simulink model "controller_ballcatcher_overdo"  (R2018b)
settings: Solver=FixedStepDiscrete  StartTime=0.0  StopTime=10.0  FixedStep=param_controller.T_a  RelTol=1e-3
InitFcn:
  | iiwa_joint_trajectoryfollowingcontrol_rigid_parameters;
values from neighbouring files (symbols this model uses):
  estimator_init_struct = struct()    [init_estimator_struct.m]
  filter_tau_p_slow_T_1 = filter_tau_slow_T_1    [parameters.m]
  filter_tau_p_T_1 = filter_tau_T_1    [parameters.m]
  filter_tau_slow_T_1 = 1./(2*pi*[200;200;200;200;200;200;200])    [parameters.m]
  filter_tau_T_1 = 1./(2*pi*[400;400;400;400;500;1000;1000])    [parameters.m]
  filter_theta_p_slow_T_1 = filter_tau_slow_T_1    [parameters.m]
  filter_theta_p_T_1 = filter_tau_T_1    [parameters.m]
  filter_theta_slow_T_1 = filter_tau_slow_T_1    [parameters.m]
  height_of_catch = 0.9    [init_estimator_struct.m]
  optitrack_data = struct()    [init_parabola.m]
  param_nullspace = struct()    [parameters.m]
  param_robot = struct()    [parameters.m]
  positions = struct()    [init_common_positions.m]
  sensor_torque_offset = [0.53;-0.095;-0.189;0.07;-0.058;0.0025;-0.12]    [parameters.m]
  timing = struct()    [parameters.m]
undefined symbols (not defined in the file or in its folder): param_controller
libraries: simulink_extras x1
(part 1 of 2)
settings Model: TCT_ExtModeMexArgs=[128 131 86 77 1 1],16842784  SimulationMode=external  Creator=cha  LastModifiedBy=user
settings SolverCC: AutoInsertRateTranBlk=on
settings DataIOCC: LoggingToFile=on  LoggingFileName=benniii.mat
settings OptimizationCC: UseFloatMulNetSlope=on  PassReuseOutputArgsThreshold=0  LocalBlockOutputs=off  EfficientFloat2IntCast=on  OptimizeBlockOrder=speed  DifferentSizesBufferReuse=on
settings DebuggingCC: ParameterTunabilityLossMsg=error
settings HardwareCC: ProdLongLongMode=on
settings ModelReferenceCC: EnableParallelModelReferenceBuilds=on  ModelReferenceNumInstancesAllowed=Single
settings SFSimCC: SimUseLocalCustomCode=off  MATLABDynamicMemAlloc=off
settings RTWCC: SystemTargetFile=TwinCAT.tlc  GenCodeOnly=on  MakeCommand=make_tct  TemplateMakefile=tct_msbuild.tmf  Description=TwinCAT Target  GenerateReport=on  RTWUseLocalCustomCode=off  TargetLang=C++
settings RTWCC: CustomHeaderCode=|
  | #define fflush(stdout)
  | #define printf(...) m_spSrv->TcReportLog(ADSLOG_MSGTYPE_LOG,__VA_ARGS__)
settings CodeAppCC: ForceParamTrailComments=on  MaxIdLength=47  OperatorAnnotations=on  StateflowObjectComments=on  MATLABSourceComments=on
settings STFCustomTargetCC: TargetLangStandard=C++03 (ISO)  CompOptLevelCompliant=on  MATLABClassNameForMDSCustomization=Simulink.SoftwareTarget.TargetSpecificTriggerConfigurationBase  GRTInterface=on  SystemTargetFile=TwinCAT.tlc

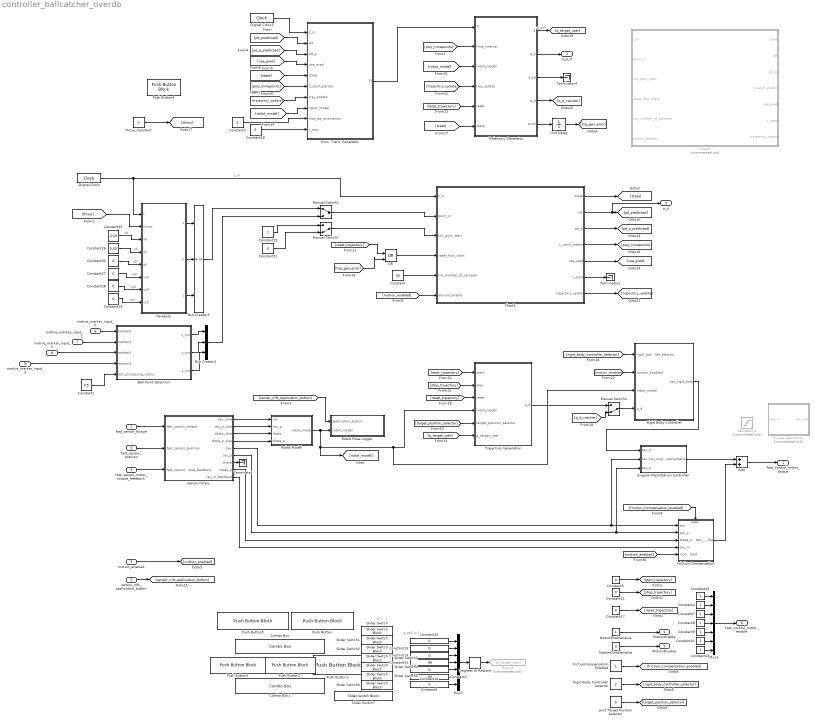
== system controller_ballcatcher_overdo ==
  note: O
  note: q_soll in °
  note: I
  fast_sensor_torque : Inport
  fast_sensor_position : Inport  Port=2
  fast_sensor_motor_torque_feedback : Inport  Port=3
  motion_enabled : Inport  Port=4
  sensor_mft_application_button : Inport  Port=5
  motive_marker_input_0 : Inport  Port=6  OutDataTypeStr=Bus: Marker
  motive_marker_input_1 : Inport  Port=7  OutDataTypeStr=Bus: Marker
  motive_marker_input_2 : Inport  Port=8  OutDataTypeStr=Bus: Marker
  motive_marker_input_3 : Inport  Port=9  OutDataTypeStr=Bus: Marker
  Add : Sum
  Ball Point Selection : MATLAB Function  TreatAsAtomicUnit=on
  Bus Creator1 : BusCreator  Inputs=3
  Bus Creator3 : BusCreator  Inputs=3
  Chart1 : Stateflow chart  TreatAsAtomicUnit=on
  Chart3 : Subsystem  Commented=on
      mask help: Simulink:masks:GenSFuncDesc_MD
      mask Help: eval('feval(''rtwprivate'',''rtwhelpview'',''rtw_sfcn_block'')');
  Combo Box : ComboBox  WebBlockId=803  SelectedLabel=2: Joint-based E/A Linearization
      settings: Values={{'1: Gravity Compensation q-based', '2: Joint-based E/A Linearization'}, [1 2]}
  Combo Box1 : ComboBox  WebBlockId=804  SelectedLabel=0: Candle position
      settings: Values={{'0: Candle position', '1: User defined position'}, [0 1]}
  Constant : Constant  Value=50
  Constant1 : Constant  Value=3.5
  Constant{4,7..10,19,22..23} (8 alike) : Constant
  Constant{3,5..6,11..14,16..17,21,27..30} (14 alike) : Constant  Value=0
  Constant15 : Constant  Value=-90
  Constant18 : Constant  Value=5
  Constant2 : Constant  Value=-90
  Constant25 : Constant  Value=-0.05
  Constant26 : Constant  Value=0.35
  Degrees to Radians : simulink_extras/Transformations/Degrees to Radians
  Digital Clock : DigitalClock  SampleTime=timing.T_optitrack
  Digital Clock1 : DigitalClock  SampleTime=timing.T_iiwa
  FictionCompensationEnabled : Constant
  Friction Compensation : Subsystem
  Goto11 : Goto  Commented=on  GotoTag=q_target_user
  Hom. Trans. Generator : MATLAB Function  TreatAsAtomicUnit=on
  Joint Target Position Selector : Constant  Value=0  OutDataTypeStr=uint32
  Manual Switch2 : ManualSwitch
  Manual Switch4 : ManualSwitch  CurrentSetting=0
  Manual Switch7 : ManualSwitch  CurrentSetting=0
  MotionDisableValue : Constant  Value=0
  MotionEnableValue : Constant
  Mux1 : Mux  Inputs=7
  Mux3 : Mux  Inputs=7
  OR : Logic  Operator=OR  IconShape=distinctive  AllPortsSameDT=off  OutDataTypeStr=boolean
  Parabola : MATLAB Function  TreatAsAtomicUnit=on
  Push Button : PushButtonBlock  WebBlockId=1354  ButtonText=Motion disable
  Push Button1 : PushButtonBlock  WebBlockId=1355  ButtonText=Reset Trajectory
  Push Button2 : PushButtonBlock  WebBlockId=1030  ButtonText=Stop trajectory
  Push Button3 : PushButtonBlock  WebBlockId=1026  ButtonText=Start trajectory
  Push Button4 : PushButtonBlock  WebBlockId=2019  ButtonText=Throw
  Push Button5 : PushButtonBlock  WebBlockId=1353  ButtonText=Motion enable
  Rigid Body Controller : Subsystem
  Rigid Body Controller Selector : Constant  Value=2  OutDataTypeStr=uint32
  Robot Model : MATLAB Function  TreatAsAtomicUnit=on
  Robot Pose Logger : MATLAB Function  TreatAsAtomicUnit=on
  Saturation1 : Saturate  Commented=on  UpperLimit=param_robot.tau_saturation_max  LowerLimit=-param_robot.tau_saturation_max
  Sensor Filters : Subsystem
  Singular Perturbation Controller : MATLAB Function  TreatAsAtomicUnit=on
  Slider Switch : SliderSwitchBlock  WebBlockId=1027  LabelPosition=Hide
      settings: Values={{'Axis1', ''}, [0 1]}
  Slider Switch1 : SliderSwitchBlock  WebBlockId=1029  LabelPosition=Hide
      settings: Values={{'Axis2', ''}, [0 1]}
  Slider Switch2 : SliderSwitchBlock  WebBlockId=1031  LabelPosition=Hide
      settings: Values={{'Axis3', ''}, [0 1]}
  Slider Switch3 : SliderSwitchBlock  WebBlockId=1022  LabelPosition=Hide
      settings: Values={{'Axis4', ''}, [0 1]}
  Slider Switch4 : SliderSwitchBlock  WebBlockId=1028  LabelPosition=Hide
      settings: Values={{'Axis5', ''}, [0 1]}
  Slider Switch5 : SliderSwitchBlock  WebBlockId=1025  LabelPosition=Hide
      settings: Values={{'Axis6', ''}, [0 1]}
  Slider Switch6 : SliderSwitchBlock  WebBlockId=1021  LabelPosition=Hide
      settings: Values={{'Axis7', ''}, [0 1]}
  Slider Switch7 : SliderSwitchBlock  WebBlockId=1032  LabelPosition=Hide
      settings: Values={{'Friction Compensation', ''}, [0 1]}
  Terminator : Terminator
  Terminator1 : Terminator
  Terminator4 : Terminator
  Throw_Constant : Constant  Value=0
  Torque Saturation1 : MATLAB Function  Commented=on  TreatAsAtomicUnit=on
  Trajectory Generation : Subsystem
  Trajectory Generator : MATLAB Function  TreatAsAtomicUnit=on
  Unit Delay : UnitDelay  SampleTime=-1
  fast_control_motor_torque : Outport
  q_p_d : Outport  Port=2  VectorParamsAs1DForOutWhenUnconnected=on
  p_d : Outport  Port=3  VectorParamsAs1DForOutWhenUnconnected=on
  MotionEnable : Outport  Port=4
  MotionDisable : Outport  Port=5
  fast_control_motor_enable : Outport  Port=6
  wires:
  MotionEnableValue/1 -> MotionEnable/1
  motion_enabled/1 -> [motion_enabled]
  MotionDisableValue/1 -> MotionDisable/1
  Sensor Filters/5(tau) -> Singular Perturbation Controller/2(tau), Friction Compensation/1(tau)
  Mux1/1 -> fast_control_motor_enable/1
  Constant22/1 -> Mux1/1
  Constant4/1 -> Mux1/2
  Constant7/1 -> Mux1/3
  Constant8/1 -> Mux1/4
  Constant9/1 -> Mux1/5
  Constant10/1 -> Mux1/6
  Constant23/1 -> Mux1/7
  fast_sensor_torque/1 -> Sensor Filters/1(fast_sensor_torque)
  fast_sensor_position/1 -> Sensor Filters/2(fast_sensor_position)
  fast_sensor_motor_torque_feedback/1 -> Sensor Filters/3(fast_sensor_motor_torque_feedback)
  Sensor Filters/9(tau_m_feedback) -> Friction Compensation/4(tau_m)
  Sensor Filters/6(tau_p) -> Singular Perturbation Controller/3(tau_p), Friction Compensation/2(tau_p)
  Sensor Filters/8(theta_p) -> Friction Compensation/3(theta_p)
  Friction Compensation/1(tau_fm_hat) -> Add/2
  Constant5/1 -> [start_trajectory]
  [motion_enabled] -> Friction Compensation/5(motion_enabled)
  Rigid Body Controller Selector/1 -> [rigid_body_controller_selector]
  FictionCompensationEnabled/1 -> [friction_compensation_enabled]
  [friction_compensation_enabled] -> Friction Compensation/Enable
  Sensor Filters/7(theta) -> Terminator/1
  Joint Target Position Selector/1 -> [target_position_selector]
  Constant6/1 -> Mux3/7
  Constant12/1 -> Mux3/1
  Constant16/1 -> Mux3/5
  Mux3/1 -> Degrees to Radians/1
  Constant15/1 -> Mux3/4
  Constant13/1 -> Mux3/2
  Constant2/1 -> Mux3/6
  Constant14/1 -> Mux3/3
  Constant11/1 -> [stop_trajectory]
  sensor_mft_application_button/1 -> [sensor_mft_application_button]
  Degrees to Radians/1 -> Goto11/1
  Sensor Filters/1(tau_slow) -> Robot Model/1(tau)
  Sensor Filters/2(tau_p_slow) -> Robot Model/2(tau_p)
  Sensor Filters/3(theta_slow) -> Robot Model/3(theta)
  Sensor Filters/4(theta_p_slow) -> Robot Model/4(theta_p)
  [sensor_mft_application_button] -> Robot Pose Logger/1(application_button)
  Robot Model/1(robot_model) -> Rigid Body Controller/3(robot_model), Trajectory Generation/4(robot_model), [robot_model], Robot Pose Logger/2(robot_model)
  Trajectory Generator/1(q) -> [q_target_user]  "q_soll"
  [use_pred] -> Hom. Trans. Generator/4(use_pred)
  [pd_p_predicted] -> Hom. Trans. Generator/3(pd_p)
  [state] -> Hom. Trans. Generator/5(state)
  Trajectory Generator/2(q_p) -> q_p_d/1
  [pd_predicted] -> Hom. Trans. Generator/2(pd)
  Constant21/1 -> Manual Switch7/2
  Constant19/1 -> Manual Switch7/1
  Digital Clock1/1 -> Hom. Trans. Generator/1(t_in)
  motive_marker_input_0/1 -> Ball Point Selection/1(marker0)
  [q_target_user] -> Trajectory Generation/6(q_target_user)
  [reset_trajectory] -> Trajectory Generation/3(reset)
  [stop_trajectory] -> Trajectory Generation/2(stop)
  [target_position_selector] -> Trajectory Generation/5(target_position_selector)
  [rigid_body_controller_selector] -> Rigid Body Controller/1(rigid_body_controller_selector)
  [start_trajectory] -> Trajectory Generation/1(start)
  [motion_enabled] -> Rigid Body Controller/2(motion_enabled)
  [robot_model] -> Trajectory Generator/3(robot_model)
  Singular Perturbation Controller/1(tau_singularperturbation) -> Add/1
  Rigid Body Controller/1(tau_rigid_body) -> Singular Perturbation Controller/1(tau_d)
  [poly_timepoints] -> Trajectory Generator/2(time_interval)
  Hom. Trans. Generator/1(Tf) -> Trajectory Generator/1(Tf)
  Trajectory Generator/4(q_d) -> [q_d_catcher]
  Manual Switch7/1 -> Chart1/3(init_goto_start)
  Chart1/1(state) -> [state]
  Chart1/2(pd) -> p_d/1, [pd_predicted]
  Chart1/3(pd_p) -> [pd_p_predicted]
  Chart1/4(t_catch_predict) -> [poly_timepoints]
  Chart1/5(use_pred) -> [use_pred]
  Chart1/6(t_start) -> Terminator1/1
  Manual Switch4/1 -> Rigid Body Controller/4(q_d)
  Trajectory Generation/1(q_d) -> Manual Switch4/1
  [q_d_catcher] -> Manual Switch4/2
  Digital Clock/1 -> Chart1/1(t_in), Parabola/1(t)  "t_in"
  Ball Point Selection/1(x_out) -> Bus Creator1/1
  Ball Point Selection/2(y_out) -> Bus Creator1/2
  Ball Point Selection/3(z_out) -> Bus Creator1/3
  [throw] -> Parabola/2(throw)
  Throw_Constant/1 -> [throw]
  Parabola/3(z) -> Bus Creator3/3
  Parabola/2(y) -> Bus Creator3/2
  Parabola/1(x) -> Bus Creator3/1
  Manual Switch2/1 -> Chart1/2(point_in)
  Bus Creator3/1 -> Manual Switch2/1
  Bus Creator1/1 -> Manual Switch2/2
  Constant26/1 -> Parabola/4(y0)  "y0"
  Constant27/1 -> Parabola/6(vx0)  "vx0"
  Constant30/1 -> Parabola/5(z0)  "z0"
  Constant25/1 -> Parabola/3(x0)  "x0"
  Constant29/1 -> Parabola/8(vz0)  "vz0"
  Constant28/1 -> Parabola/7(vy0)  "vy0"
  Trajectory Generator/3(q_pp) -> Terminator4/1
  [poly_timepoints] -> Hom. Trans. Generator/6(t_catch_period)
  [trajectory_update] -> Trajectory Generator/4(traj_update)
  Chart1/7(trajectory_update) -> [trajectory_update]
  [robot_model] -> Hom. Trans. Generator/8(robot_model)
  Constant/1 -> Chart1/5(init_number_of_samples)
  [trajectory_update] -> Hom. Trans. Generator/7(traj_update)
  Constant1/1 -> Ball Point Selection/5(ball_processing_radius)
  Constant3/1 -> Hom. Trans. Generator/9(max_ee_orientation)
  [reset_trajectory] -> Trajectory Generator/5(reset)
  [motion_enabled] -> Chart1/6(motion_enable)
  Constant18/1 -> Hom. Trans. Generator/10(r_max)
  Add/1 -> fast_control_motor_torque/1
  motive_marker_input_1/1 -> Ball Point Selection/2(marker1)
  motive_marker_input_2/1 -> Ball Point Selection/3(marker2)
  motive_marker_input_3/1 -> Ball Point Selection/4(marker3)
  [state] -> Trajectory Generator/6(state)
  Constant17/1 -> [reset_trajectory]
  Trajectory Generator/5(error) -> Unit Delay/1
  Unit Delay/1 -> [traj_gen_error]
  OR/1 -> Chart1/4(reset_flow_chart)
  [reset_trajectory] -> OR/1
  [traj_gen_error] -> OR/2

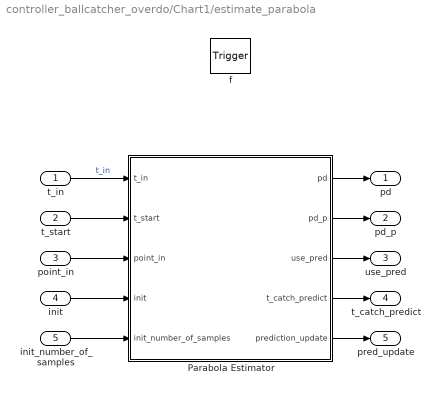
== system controller_ballcatcher_overdo/Chart1/estimate_parabola ==
  t_in : Inport  OutDataTypeStr=double  PortDimensions=1
  t_start : Inport  Port=2  OutDataTypeStr=double  PortDimensions=1
  point_in : Inport  Port=3  OutDataTypeStr=double  PortDimensions=3
  init : Inport  Port=4  OutDataTypeStr=double  PortDimensions=1
  init_number_of_samples : Inport  Port=5  OutDataTypeStr=double  PortDimensions=1
  f : TriggerPort  TriggerType=function-call  VariantControl=(inherit)
      settings: CopyFcn=Stateflow.SLINSF.SimulinkMan.removeBlockPreDeleteFcn  PreDeleteFcn=Stateflow.SLINSF.SimulinkMan.unsafePredeleteFcn
  Parabola Estimator : MATLAB Function  TreatAsAtomicUnit=on
  pd : Outport  PortDimensions=3  VectorParamsAs1DForOutWhenUnconnected=on
  pd_p : Outport  Port=2  PortDimensions=3  VectorParamsAs1DForOutWhenUnconnected=on
  use_pred : Outport  Port=3  PortDimensions=1  VectorParamsAs1DForOutWhenUnconnected=on
  t_catch_predict : Outport  Port=4  PortDimensions=[1,2]  VectorParamsAs1DForOutWhenUnconnected=on
  pred_update : Outport  Port=5  VectorParamsAs1DForOutWhenUnconnected=on
  wires:
  Parabola Estimator/2(pd_p) -> pd_p/1
  Parabola Estimator/1(pd) -> pd/1
  Parabola Estimator/4(t_catch_predict) -> t_catch_predict/1
  Parabola Estimator/3(use_pred) -> use_pred/1
  t_in/1 -> Parabola Estimator/1(t_in)  "t_in"
  point_in/1 -> Parabola Estimator/3(point_in)
  t_start/1 -> Parabola Estimator/2(t_start)
  init/1 -> Parabola Estimator/4(init)
  Parabola Estimator/5(prediction_update) -> pred_update/1
  init_number_of_samples/1 -> Parabola Estimator/5(init_number_of_samples)

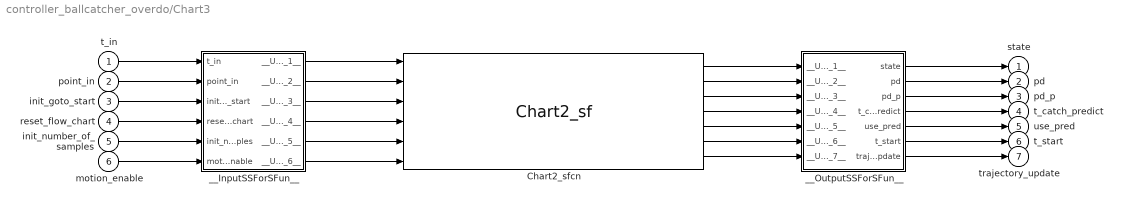
== system controller_ballcatcher_overdo/Chart3 ==
  t_in : Inport
  point_in : Inport  Port=2
  init_goto_start : Inport  Port=3
  reset_flow_chart : Inport  Port=4
  init_number_of_samples : Inport  Port=5
  motion_enable : Inport  Port=6
  Chart2_sfcn : S-Function  FunctionName=Chart2_sf  SFunctionModules=""  SFunctionDeploymentMode=off  EnableBusSupport=off  mask{rtw_sf_name=Chart2_sf, showVar=off}
      mask prompts: rtw_sf_name "Simulink:masks:GenSFuncName_MP"; showVar "Simulink:masks:GenSFuncShowModuleList_MP"
      mask help: Simulink:masks:GenSFuncDesc_MD
      mask init:
      | displist = '';
      | if ~strcmp(get_param(gcb, 'FunctionName'), rtw_sf_name);
      |   set_param(gcb, 'FunctionName', rtw_sf_name);
      | end
      | % Check if we are generating code
      | rtw_mode = false;
      | if strcmpi(get_param(bdroot(gcb),'SimulationStatus'),'Initializing')
      | 	rtw_mode = strcmpi(get_param(bdroot(gcb),'BuildingRTWCode'),'on') && ...
      | 		~strcmpi(get_param(bdroot(gcb),'TargetStyle'),'SimulationTarget');
      | end
      | if showVar || rtw_mode
      | 	if exist('rtwsfunc') == 2 | exist('rtwsfunc') == 6
      | 		tmplist = rtwsfunc(rtw_sf_name,gcb);
      | 		tmplist = DAStudio.message('Simulink:masks:GenSFuncListOfModules_IC', tmplist);
      | 	elseif showVar
      | 		tmplist1 = DAStudio.message('Simulink:masks:GenSFuncListOfModules_IC', '');
      |         tmplist2 = DAStudio.message('Simulink:masks:GenSFuncNotLicensed_IC');
      |         tmplist = [tmplist1 tmplist2];
      |  	end
      | end
      | if showVar
      |   displist = tmplist;
      | end
      settings: CopyFcn=|
      | if ~strcmp(get_param(gcb,'Linkstatus'),'none') && ...
      | ~strcmp(get_param(gcb,'Linkstatus'),'implicit')
      |   set_param(gcb,'LinkStatus','none');
      | end
      mask Help: eval('feval(''rtwprivate'',''rtwhelpview'',''rtw_sfcn_block'')');
      mask Display:
      | port_label('input',1,'t_in');
      | port_label('input',2,'point_in');
      | port_label('input',3,'init_goto_start');
      | port_label('input',4,'reset_flow_chart');
      | port_label('input',5,'init_number_of_samples');
      | port_label('input',6,'motion_enable');
      | port_label('output',1,'state');
      | port_label('output',2,'pd');
      | port_label('output',3,'pd_p');
      | port_label('output',4,'t_catch_predict');
      | port_label('output',5,'use_pred');
      | port_label('output',6,'t_start');
      | port_label('output',7,'trajectory_update');
  __InputSSForSFun__ : Subsystem
  __OutputSSForSFun__ : Subsystem
  state : Outport  VectorParamsAs1DForOutWhenUnconnected=on
  pd : Outport  Port=2  VectorParamsAs1DForOutWhenUnconnected=on
  pd_p : Outport  Port=3  VectorParamsAs1DForOutWhenUnconnected=on
  t_catch_predict : Outport  Port=4  VectorParamsAs1DForOutWhenUnconnected=on
  use_pred : Outport  Port=5  VectorParamsAs1DForOutWhenUnconnected=on
  t_start : Outport  Port=6  VectorParamsAs1DForOutWhenUnconnected=on
  trajectory_update : Outport  Port=7  VectorParamsAs1DForOutWhenUnconnected=on
  wires:
  __OutputSSForSFun__/7(trajectory_update) -> trajectory_update/1
  __OutputSSForSFun__/6(t_start) -> t_start/1
  __OutputSSForSFun__/5(use_pred) -> use_pred/1
  __OutputSSForSFun__/4(t_catch_predict) -> t_catch_predict/1
  __OutputSSForSFun__/3(pd_p) -> pd_p/1
  __OutputSSForSFun__/2(pd) -> pd/1
  __OutputSSForSFun__/1(state) -> state/1
  Chart2_sfcn/7 -> __OutputSSForSFun__/7(__UniqueInportName__7__)
  Chart2_sfcn/6 -> __OutputSSForSFun__/6(__UniqueInportName__6__)
  Chart2_sfcn/5 -> __OutputSSForSFun__/5(__UniqueInportName__5__)
  Chart2_sfcn/4 -> __OutputSSForSFun__/4(__UniqueInportName__4__)
  Chart2_sfcn/3 -> __OutputSSForSFun__/3(__UniqueInportName__3__)
  Chart2_sfcn/2 -> __OutputSSForSFun__/2(__UniqueInportName__2__)
  Chart2_sfcn/1 -> __OutputSSForSFun__/1(__UniqueInportName__1__)
  __InputSSForSFun__/6(__UniqueOutportName__6__) -> Chart2_sfcn/6
  __InputSSForSFun__/5(__UniqueOutportName__5__) -> Chart2_sfcn/5
  __InputSSForSFun__/4(__UniqueOutportName__4__) -> Chart2_sfcn/4
  __InputSSForSFun__/3(__UniqueOutportName__3__) -> Chart2_sfcn/3
  __InputSSForSFun__/2(__UniqueOutportName__2__) -> Chart2_sfcn/2
  __InputSSForSFun__/1(__UniqueOutportName__1__) -> Chart2_sfcn/1
  motion_enable/1 -> __InputSSForSFun__/6(motion_enable)
  init_number_of_samples/1 -> __InputSSForSFun__/5(init_number_of_samples)
  reset_flow_chart/1 -> __InputSSForSFun__/4(reset_flow_chart)
  init_goto_start/1 -> __InputSSForSFun__/3(init_goto_start)
  point_in/1 -> __InputSSForSFun__/2(point_in)
  t_in/1 -> __InputSSForSFun__/1(t_in)

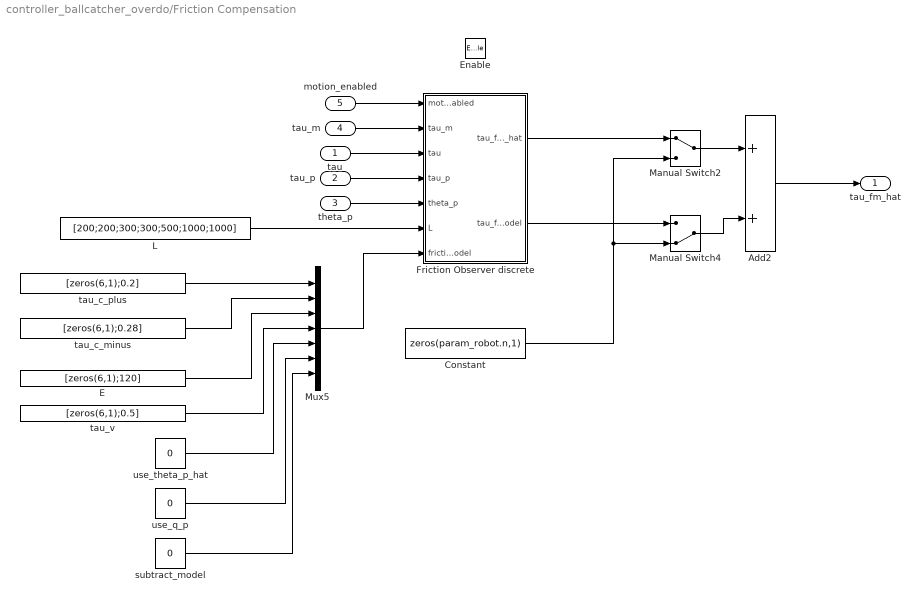
== system controller_ballcatcher_overdo/Friction Compensation ==
  tau : Inport
  tau_p : Inport  Port=2
  theta_p : Inport  Port=3
  tau_m : Inport  Port=4
  motion_enabled : Inport  Port=5
  Enable : EnablePort
  Add2 : Sum
  Constant : Constant  Value=zeros(param_robot.n,1)
  E : Constant  Value=[zeros(6,1);120]
  Friction Observer discrete : MATLAB Function  TreatAsAtomicUnit=on
  L : Constant  Value=[200;200;300;300;500;1000;1000]
  Manual Switch2 : ManualSwitch
  Manual Switch4 : ManualSwitch  CurrentSetting=0
  Mux5 : Mux  Inputs=7
  subtract_model : Constant  Value=0
  tau_c_minus : Constant  Value=[zeros(6,1);0.28]
  tau_c_plus : Constant  Value=[zeros(6,1);0.2]
  tau_v : Constant  Value=[zeros(6,1);0.5]
  use_q_p : Constant  Value=0
  use_theta_p_hat : Constant  Value=0
  tau_fm_hat : Outport
  wires:
  tau_p/1 -> Friction Observer discrete/4(tau_p)
  L/1 -> Friction Observer discrete/6(L)
  subtract_model/1 -> Mux5/7
  Friction Observer discrete/2(tau_f_model) -> Manual Switch4/1
  Manual Switch2/1 -> Add2/1
  tau_m/1 -> Friction Observer discrete/2(tau_m)
  use_q_p/1 -> Mux5/6
  Manual Switch4/1 -> Add2/2
  Friction Observer discrete/1(tau_fm_hat) -> Manual Switch2/1
  tau_c_minus/1 -> Mux5/2
  tau_v/1 -> Mux5/4
  use_theta_p_hat/1 -> Mux5/5
  Add2/1 -> tau_fm_hat/1
  Mux5/1 -> Friction Observer discrete/7(friction_model)
  motion_enabled/1 -> Friction Observer discrete/1(motion_enabled)
  tau_c_plus/1 -> Mux5/1
  theta_p/1 -> Friction Observer discrete/5(theta_p)
  Constant/1 -> Manual Switch4/2, Manual Switch2/2
  tau/1 -> Friction Observer discrete/3(tau)
  E/1 -> Mux5/3

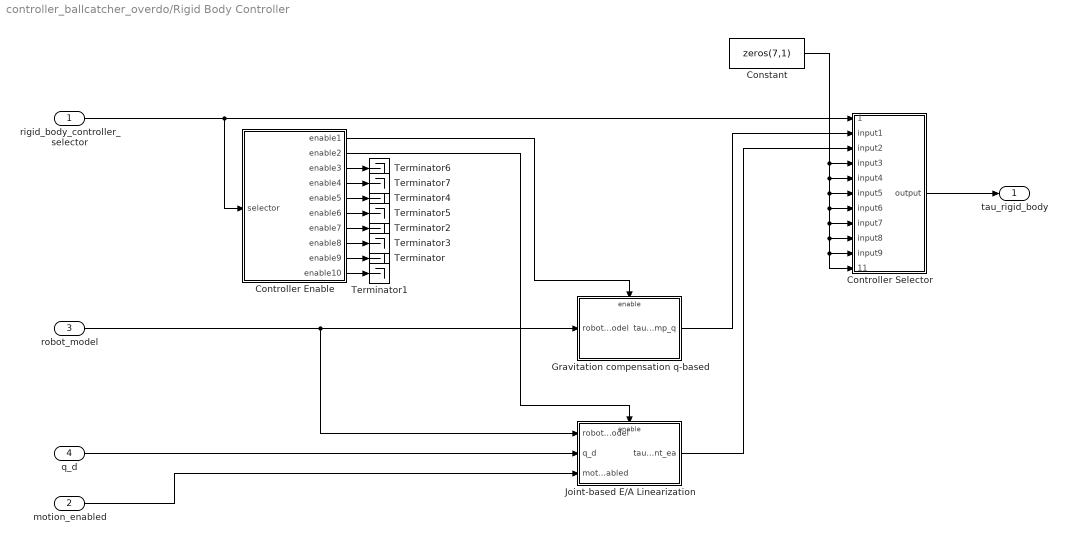
== system controller_ballcatcher_overdo/Rigid Body Controller ==
  rigid_body_controller_selector : Inport
  motion_enabled : Inport  Port=2
  robot_model : Inport  Port=3
  q_d : Inport  Port=4
  Constant : Constant  Value=zeros(7,1)
  Controller Enable : MATLAB Function  TreatAsAtomicUnit=on
  Controller Selector : MATLAB Function  TreatAsAtomicUnit=on
  Gravitation compensation q-based : Subsystem
  Joint-based E/A Linearization : Subsystem
  Terminator{,1..7} (8 alike) : Terminator
  tau_rigid_body : Outport
  wires:
  Controller Selector/1(output) -> tau_rigid_body/1
  rigid_body_controller_selector/1 -> Controller Selector/1(selector), Controller Enable/1(selector)
  robot_model/1 -> Gravitation compensation q-based/1(robot_model), Joint-based E/A Linearization/1(robot_model)
  Gravitation compensation q-based/1(tau_d_gravcomp_q) -> Controller Selector/2(input1)
  Controller Enable/1(enable1) -> Gravitation compensation q-based/Enable
  q_d/1 -> Joint-based E/A Linearization/2(q_d)
  motion_enabled/1 -> Joint-based E/A Linearization/3(motion_enabled)
  Joint-based E/A Linearization/1(tau_d_joint_ea) -> Controller Selector/3(input2)
  Controller Enable/2(enable2) -> Joint-based E/A Linearization/Enable
  Controller Enable/9(enable9) -> Terminator/1
  Controller Enable/10(enable10) -> Terminator1/1
  Controller Enable/7(enable7) -> Terminator2/1
  Controller Enable/8(enable8) -> Terminator3/1
  Controller Enable/6(enable6) -> Terminator5/1
  Controller Enable/4(enable4) -> Terminator7/1
  Controller Enable/5(enable5) -> Terminator4/1
  Constant/1 -> Controller Selector/4(input3), Controller Selector/11(input10), Controller Selector/10(input9), Controller Selector/9(input8), Controller Selector/8(input7), Controller Selector/7(input6), Controller Selector/6(input5), Controller Selector/5(input4)
  Controller Enable/3(enable3) -> Terminator6/1

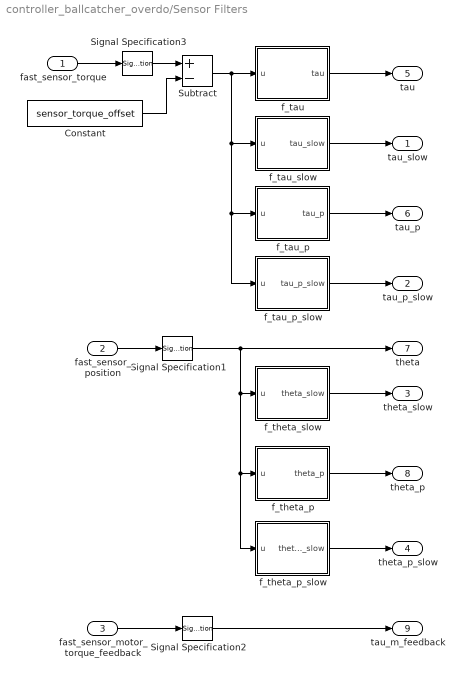
== system controller_ballcatcher_overdo/Sensor Filters ==
  fast_sensor_torque : Inport
  fast_sensor_position : Inport  Port=2
  fast_sensor_motor_torque_feedback : Inport  Port=3
  Constant : Constant  Value=sensor_torque_offset
  Signal Specification1 : SignalSpecification  Dimensions=7
  Signal Specification2 : SignalSpecification  Dimensions=7
  Signal Specification3 : SignalSpecification  Dimensions=7
  Subtract : Sum  Inputs=+-
  f_tau : MATLAB Function  TreatAsAtomicUnit=on
  f_tau_p : MATLAB Function  TreatAsAtomicUnit=on
  f_tau_p_slow : MATLAB Function  TreatAsAtomicUnit=on
  f_tau_slow : MATLAB Function  TreatAsAtomicUnit=on
  f_theta_p : MATLAB Function  TreatAsAtomicUnit=on
  f_theta_p_slow : MATLAB Function  TreatAsAtomicUnit=on
  f_theta_slow : MATLAB Function  TreatAsAtomicUnit=on
  tau_slow : Outport
  tau_p_slow : Outport  Port=2
  theta_slow : Outport  Port=3
  theta_p_slow : Outport  Port=4
  tau : Outport  Port=5
  tau_p : Outport  Port=6
  theta : Outport  Port=7
  theta_p : Outport  Port=8
  tau_m_feedback : Outport  Port=9
  wires:
  fast_sensor_position/1 -> Signal Specification1/1
  fast_sensor_motor_torque_feedback/1 -> Signal Specification2/1
  f_theta_p/1(theta_p) -> theta_p/1
  Signal Specification1/1 -> theta/1, f_theta_slow/1(u), f_theta_p_slow/1(u), f_theta_p/1(u)
  f_tau_p/1(tau_p) -> tau_p/1
  f_theta_p_slow/1(theta_p_slow) -> theta_p_slow/1
  f_tau/1(tau) -> tau/1
  Signal Specification2/1 -> tau_m_feedback/1
  f_theta_slow/1(theta_slow) -> theta_slow/1
  f_tau_slow/1(tau_slow) -> tau_slow/1
  f_tau_p_slow/1(tau_p_slow) -> tau_p_slow/1
  Constant/1 -> Subtract/2
  Subtract/1 -> f_tau/1(u), f_tau_slow/1(u), f_tau_p_slow/1(u), f_tau_p/1(u)
  fast_sensor_torque/1 -> Signal Specification3/1
  Signal Specification3/1 -> Subtract/1

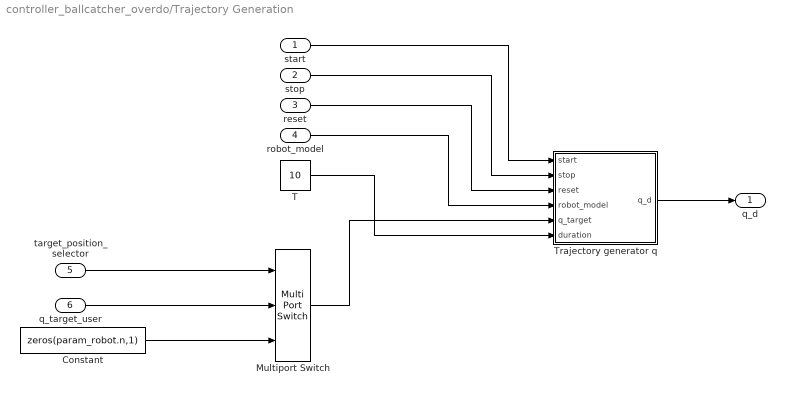
== system controller_ballcatcher_overdo/Trajectory Generation ==
  start : Inport
  stop : Inport  Port=2
  reset : Inport  Port=3
  robot_model : Inport  Port=4
  target_position_selector : Inport  Port=5
  q_target_user : Inport  Port=6
  Constant : Constant  Value=zeros(param_robot.n,1)
  Multiport Switch : MultiPortSwitch  Inputs=2  DiagnosticForDefault=None
  T : Constant  Value=10
  Trajectory generator q : MATLAB Function  TreatAsAtomicUnit=on
  q_d : Outport
  wires:
  start/1 -> Trajectory generator q/1(start)
  reset/1 -> Trajectory generator q/3(reset)
  T/1 -> Trajectory generator q/6(duration)
  stop/1 -> Trajectory generator q/2(stop)
  robot_model/1 -> Trajectory generator q/4(robot_model)
  Constant/1 -> Multiport Switch/3
  q_target_user/1 -> Multiport Switch/2
  Multiport Switch/1 -> Trajectory generator q/5(q_target)
  target_position_selector/1 -> Multiport Switch/1
  Trajectory generator q/1(q_d) -> q_d/1

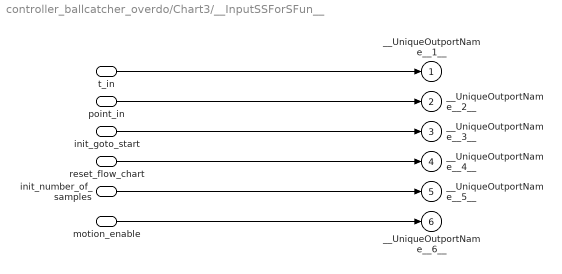
== system controller_ballcatcher_overdo/Chart3/__InputSSForSFun__ ==
  t_in : Inport
  point_in : Inport  Port=2
  init_goto_start : Inport  Port=3
  reset_flow_chart : Inport  Port=4
  init_number_of_samples : Inport  Port=5
  motion_enable : Inport  Port=6
  __UniqueOutportName__1__ : Outport
  __UniqueOutportName__2__ : Outport  Port=2
  __UniqueOutportName__3__ : Outport  Port=3
  __UniqueOutportName__4__ : Outport  Port=4
  __UniqueOutportName__5__ : Outport  Port=5
  __UniqueOutportName__6__ : Outport  Port=6
  wires:
  motion_enable/1 -> __UniqueOutportName__6__/1
  init_number_of_samples/1 -> __UniqueOutportName__5__/1
  reset_flow_chart/1 -> __UniqueOutportName__4__/1
  init_goto_start/1 -> __UniqueOutportName__3__/1
  point_in/1 -> __UniqueOutportName__2__/1
  t_in/1 -> __UniqueOutportName__1__/1

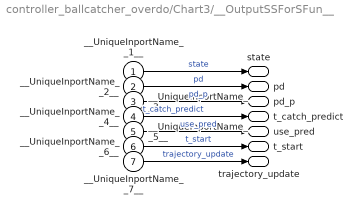
== system controller_ballcatcher_overdo/Chart3/__OutputSSForSFun__ ==
  __UniqueInportName__1__ : Inport
  __UniqueInportName__2__ : Inport  Port=2
  __UniqueInportName__3__ : Inport  Port=3
  __UniqueInportName__4__ : Inport  Port=4
  __UniqueInportName__5__ : Inport  Port=5
  __UniqueInportName__6__ : Inport  Port=6
  __UniqueInportName__7__ : Inport  Port=7
  state : Outport  VectorParamsAs1DForOutWhenUnconnected=on
  pd : Outport  Port=2  VectorParamsAs1DForOutWhenUnconnected=on
  pd_p : Outport  Port=3  VectorParamsAs1DForOutWhenUnconnected=on
  t_catch_predict : Outport  Port=4  VectorParamsAs1DForOutWhenUnconnected=on
  use_pred : Outport  Port=5  VectorParamsAs1DForOutWhenUnconnected=on
  t_start : Outport  Port=6  VectorParamsAs1DForOutWhenUnconnected=on
  trajectory_update : Outport  Port=7  VectorParamsAs1DForOutWhenUnconnected=on
  wires:
  __UniqueInportName__7__/1 -> trajectory_update/1  "trajectory_update"
  __UniqueInportName__6__/1 -> t_start/1  "t_start"
  __UniqueInportName__5__/1 -> use_pred/1  "use_pred"
  __UniqueInportName__4__/1 -> t_catch_predict/1  "t_catch_predict"
  __UniqueInportName__3__/1 -> pd_p/1  "pd_p"
  __UniqueInportName__2__/1 -> pd/1  "pd"
  __UniqueInportName__1__/1 -> state/1  "state"

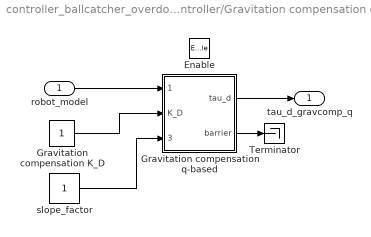
== system controller_ballcatcher_overdo/Rigid Body Controller/Gravitation compensation q-based ==
  robot_model : Inport
  Enable : EnablePort  StatesWhenEnabling=reset
  Gravitation compensation q-based : MATLAB Function  TreatAsAtomicUnit=on
  Gravitation compensation K_D : Constant
  Terminator : Terminator
  slope_factor : Constant
  tau_d_gravcomp_q : Outport
  wires:
  robot_model/1 -> Gravitation compensation q-based/1(robot_model)
  Gravitation compensation q-based/1(tau_d) -> tau_d_gravcomp_q/1
  Gravitation compensation K_D/1 -> Gravitation compensation q-based/2(K_D)
  Gravitation compensation q-based/2(barrier) -> Terminator/1
  slope_factor/1 -> Gravitation compensation q-based/3(slope_factor)

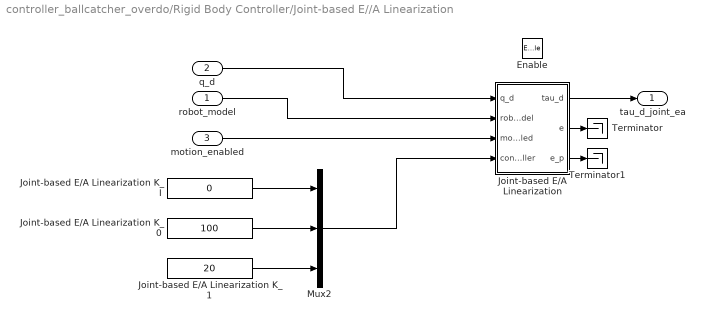
== system controller_ballcatcher_overdo/Rigid Body Controller/Joint-based E//A Linearization ==
  robot_model : Inport
  q_d : Inport  Port=2
  motion_enabled : Inport  Port=3
  Enable : EnablePort  StatesWhenEnabling=reset
  Joint-based E/A Linearization : MATLAB Function  TreatAsAtomicUnit=on
  Joint-based E/A Linearization K_0 : Constant  Value=100
  Joint-based E/A Linearization K_1 : Constant  Value=20
  Joint-based E/A Linearization K_I : Constant  Value=0
  Mux2 : Mux  Inputs=3
  Terminator : Terminator
  Terminator1 : Terminator
  tau_d_joint_ea : Outport
  wires:
  motion_enabled/1 -> Joint-based E/A Linearization/3(motion_enabled)
  Joint-based E/A Linearization K_I/1 -> Mux2/1
  Joint-based E/A Linearization K_1/1 -> Mux2/3
  Joint-based E/A Linearization K_0/1 -> Mux2/2
  Joint-based E/A Linearization/1(tau_d) -> tau_d_joint_ea/1
  q_d/1 -> Joint-based E/A Linearization/1(q_d)
  Mux2/1 -> Joint-based E/A Linearization/4(controller)
  robot_model/1 -> Joint-based E/A Linearization/2(robot_model)
  Joint-based E/A Linearization/2(e) -> Terminator/1
  Joint-based E/A Linearization/3(e_p) -> Terminator1/1

== matlab function controller_ballcatcher_overdo/Parabola ==
  data: t input; x output; y output; z output; throw input; x0 input; y0 input; z0 input; vx0 input; vy0 input; vz0 input; optitrack_data parameter; param_controller parameter; timing parameter
function [x,y,z] = fcn(t,throw,x0,y0,z0,vx0,vy0,vz0,optitrack_data,param_controller,timing)
  
%   persistent t_throw_start throw_pers;
% 
%   if(isempty(t_throw_start))
%     t_throw_start=0;
%     throw_pers = 0;
%   end
%   
%   x = 0;
%   y = 0;
%   z = 0;
% 
%   if(throw)
%     t_throw_start = t+timing.T_optitrack;
%     throw_pers = 1;
%   end
%   
%   if(throw_pers && throw==0)
%     t_diff = t - t_throw_start;
% 
%     x = x0 + vx0*t_diff;
%     y = y0 + vy0*t_diff;
%     z = z0 + vz0*t_diff - (param_controller.g/2)*t_diff.^2;
%     
%     if z < (0.7)
%       throw_pers = 0;
%     end
%   end
  
  persistent t_throw_start throw_pers i;

  if(isempty(t_throw_start))
    t_throw_start=0;
    throw_pers = 0;
    i = 1;
  end
  
  x = 0;
  y = 0;
  z = 0;

  if(throw)
    t_throw_start = t+timing.T_optitrack;
    throw_pers = 1;
    i = 1;
  end
  
  if(throw_pers && throw==0)
    x = optitrack_data.x(i) + x0;
    y = optitrack_data.y(i) + y0;
    z = optitrack_data.z(i) + z0;
    
    i = i+1;
    
    if z < (0.7)
      throw_pers = 0;
    end
  end
end

== matlab function controller_ballcatcher_overdo/Ball Point Selection ==
  data: marker0 input; marker1 input; marker2 input; marker3 input; x_out output; y_out output; z_out output; ball_processing_radius input
function [x_out,y_out,z_out] = fcn(marker0,marker1,marker2,marker3,ball_processing_radius)
  persistent ballId;
  
  if isempty(ballId)
    ballId = int16(0);
  end
  
  x = marker0.x;
  y = marker0.y;
  z = marker0.z;
  
  if ((ballId == 0) && ((x ~= 0) || (y ~= 0) || (z ~= 0)))
    ballId = marker0.MarkerID;
    fprintf('found marker0 for the first time!');
    fprintf('Marker0 ID: %i',marker0.MarkerID);
  elseif (ballId ~= 0)
    if marker1.MarkerID == ballId
      x = marker1.x;
      y = marker1.y;
      z = marker1.z;
      fprintf('switched to marker 1');
    elseif marker2.MarkerID == ballId
      x = marker2.x;
      y = marker2.y;
      z = marker2.z;
      fprintf('switched to marker 2');
    elseif marker3.MarkerID == ballId
      x = marker3.x;
      y = marker3.y;
      z = marker3.z;
      fprintf('switched to marker 3');
    end
  end
  
  r = sqrt(x^2+y^2);
  if(r > ball_processing_radius)
    x_out = 0;
    y_out = 0;
    z_out = 0;
  else
    x_out = x;
    y_out = y;
    z_out = z;
  end
end

== matlab function controller_ballcatcher_overdo/Sensor Filters/f_tau ==
  data: u input; tau output; param_controller parameter; filter_tau_T_1 parameter
function tau = func(u,param_controller, filter_tau_T_1)
  persistent x;
  
  T_1=filter_tau_T_1;
  alpha=exp(-param_controller.T_a./T_1);
  if(isempty(x))
    x=1./(1-alpha).*u;
    tau=u;
  else
    tau=(1-alpha).*x;
    x=alpha.*x+u;
  end
end

== matlab function controller_ballcatcher_overdo/Sensor Filters/f_tau_p ==
  data: u input; tau_p output; filter_tau_p_T_1 parameter; param_controller parameter
function tau_p = func(u,filter_tau_p_T_1,param_controller)
  persistent x;
  
  T_1=filter_tau_p_T_1;
  V=1/param_controller.T_a*(1-exp(-param_controller.T_a./T_1));
  if(isempty(x))
    x=-V.*u;
    tau_p=zeros(size(u));
  else
    tau_p=x+V.*u;
    x=exp(-param_controller.T_a./T_1).*x+(exp(-param_controller.T_a./T_1)-1).*V.*u;
  end
end

== matlab function controller_ballcatcher_overdo/Singular Perturbation Controller ==
  data: tau_d input; tau input; tau_p input; tau_singularperturbation output; param_controller parameter
function tau_singularperturbation  = fcn(tau_d,tau,tau_p,param_controller)
  %Implementation is taken from Ott 2008, chapter 5.4.
  tau_singularperturbation_controller_K=-param_controller.singular_perturbation.K_tau.*(tau-tau_d);
  tau_singularperturbation_controller_D=-param_controller.singular_perturbation.D_tau.*tau_p;
  tau_singularperturbation_controller=tau_singularperturbation_controller_K...
    +tau_singularperturbation_controller_D;
  tau_singularperturbation=tau_d+tau_singularperturbation_controller;
end

== matlab function controller_ballcatcher_overdo/Trajectory Generator ==
  data: q output; Tf input; time_interval input; q_p output; q_pp output; param_robot parameter; q_d output; robot_model input; positions parameter; traj_update input; timing parameter; reset input; state input; error output size=1
function [q,q_p,q_pp,q_d,error]  = fcn(Tf,time_interval,param_robot,robot_model,positions,traj_update,timing,reset,state)
    persistent q0 q0_p q0_pp qf T_0 T_f q_ q_p_ q_pp_ t_ started error_;
    
    n = 7;
    qf_p = zeros(n,1);
    qf_pp = zeros(n,1);
    
    if isempty(q0)
      q0 = robot_model.q;
      q0_p = zeros(n,1);
      q0_pp = zeros(n,1);
      qf = robot_model.q;
      T_0 = 0;
      T_f = 0;
      q_ = robot_model.q;
      q_p_ = zeros(n,1);
      q_pp_ = zeros(n,1);
      t_ = 0;
      started = false;
      error_ = false;
    end
    
    if traj_update || reset
       q0 = q_;
       q0_p = q_p_;
       q0_pp = q_pp_;
        
       if reset
         qf = robot_model.q;
         T_0 = 0;
         T_f = 0;
         started = false;
       else
         if isequal(Tf,positions.T_candle)
            qf = zeros(n,1);
         else
            % if state==2 -> search for inv. kin. solution which is nearest
            % to current robot configuration
            [~,qf,~]=inverse_kinematics_analytic_schweng(Tf,param_robot,state==2,q_);
         end
         T_0 = time_interval(1);
         T_f = time_interval(2);
         started = true;
       end
       
       t_ = 0;
    end
    
    if reset
      error_ = false;
    end
    
    T = T_f-T_0;
    
    H = robot_model.H;
    x_ee = H(1,4);
    y_ee = H(2,4);
    z_ee = H(3,4);
    
    % safety check: check if EE moves to far from starting position
    if (state == 2 && (x_ee < 0.2 || abs(y_ee) > 0.5 || z_ee > 1))
      error_ = true;
      started = false;
      fprintf('Error in Trajectory Generation: Endeffector out of operational space.');
    end
    
    if error_
        started = false;
    elseif t_ < 0
        started = false;
        q_d_temp=[q0;zeros(size(q0));zeros(size(q0))];
        q_ = q_d_temp(1:7);
        q_p_ = q_d_temp(8:14);
        q_pp_ = q_d_temp(15:21);
    elseif(t_>=T)
        started = false;
        q_d_temp=[qf;zeros(size(qf));zeros(size(qf))];
        q_ = q_d_temp(1:7);
        q_p_ = q_d_temp(8:14);
        q_pp_ = q_d_temp(15:21);
    elseif started
        t0 = 0;
        tf = T;

        for i = 1:n
            A = [1,t0,(t0^2)/2,(t0^3)/6,(t0^4)/24,(t0^5)/120;...
                1,tf,(tf^2)/2,(tf^3)/6,(tf^4)/24,(tf^5)/120;...
                0,1,t0,(t0^2)/2,(t0^3)/6,(t0^4)/24;...
                0,1,tf,(tf^2)/2,(tf^3)/6,(tf^4)/24;...
                0,0,1,t0,(t0^2)/2,(t0^3)/6;...
                0,0,1,tf,(tf^2)/2,(tf^3)/6];

            coeffs = (A\[q0(i);qf(i);q0_p(i);qf_p(i);q0_pp(i);qf_pp(i)])';
            
            p = flip(coeffs);
            % take factorials into account to match initial equations
            p(1) = p(1)/120;
            p(2) = p(2)/24;
            p(3) = p(3)/6;
            p(4) = p(4)/2;
            
            q_(i) = polyval(p,t_);
            
            pd = polyder(p);
            q_p_(i) = polyval(pd,t_);
            
            pdd = polyder(pd);
            q_pp_(i) = polyval(pdd,t_);
            
            % safety check: check if q_p exceeds velocity limits
            q_pp_roots = roots(pdd);
            q_p_extrema = polyval(pd,q_pp_roots);
            pddd = polyder(pdd);

            for z=1:size(q_p_extrema,1)
              if polyval(pddd,q_pp_roots(z))~=0 &&...
                  q_pp_roots(z)<=tf &&...
                  q_pp_roots(z)>=t0 &&...
                  (q_p_extrema(z)>=param_robot.q_p_limit_upper(i) ||...
                  q_p_extrema(z)<=param_robot.q_p_limit_lower(i))
                error_ = true;
                started = false;
                fprintf('Error in Trajectory Generation: Planned trajectory exceeds joint velocitiy limits in Axis %i', int8(i));
                break;
              end
            end
        end    
    end
    
    q = q_;
    q_p = q_p_;
    q_pp = q_pp_;
    
    q_d = zeros(3*n,1);
    q_d(1:n)=q;
    q_d(n+1:2*n)=q_p;
    q_d(2*n+1:3*n)=q_pp;
    
    if started
       t_ = t_ + timing.T_iiwa; 
    else
        %Hold last position, set velocity and acceleration zero
        q_d(n+1:end)=0;
    end
    
    error = error_;
        
    q_p = rad2deg(q_p);

== matlab function controller_ballcatcher_overdo/Hom. Trans. Generator ==
  data: t_in input; pd input; pd_p input; Tf output; use_pred input; state input; t_catch_period input; traj_update input; robot_model input; max_ee_orientation input; r_max input
function Tf   = trajectory_generator(t_in,pd,pd_p,use_pred,state,t_catch_period,traj_update,robot_model,max_ee_orientation,r_max)
    [Tf]=ball_follow_trajectory(pd,pd_p,use_pred,state,t_catch_period,t_in,traj_update,robot_model.H,max_ee_orientation,r_max);
end

== stateflow chart controller_ballcatcher_overdo/Chart1 ==
  state [pd,pd_p,use_pred,t_catch_predict,pred_update] = estimate_parabola(t_in,t_start,point_in,init,init_number_of_samples) [function]
  state INIT
    entry:
    state=0;
    use_pred=0;
    trajectory_update = 0;
    t_catch_predict=[0,0];
    %pd=positions.candle;
    %pd_p=positions.candle_p;
  state INIT_GOTO_START
    entry:
    trajectory_update = 1;
    t_catch_predict=[t_in,t_in+0.5];
    pd=positions.start;
    pd_p=positions.start_p;
    during:
    trajectory_update = 0;
  state READY
    entry:
    state=1;
    trajectory_update = 0;
  state CATCH
    entry:
    state=2;
    t_start=t_in;
    [pd,pd_p,use_pred,t_catch_predict,trajectory_update] = estimate_parabola(t_in,t_in,point_in,1,init_number_of_samples);
    during:
    [pd,pd_p,use_pred,t_catch_predict,trajectory_update] = estimate_parabola(t_in,t_start,point_in,0,init_number_of_samples);
    exit:
    use_pred=0;
    trajectory_update = 0;
  state GO_TO_START_FROM_NO_CATCH
    entry:
    trajectory_update = 1;
    state=4;
    t_catch_predict=[t_in,t_in+0.5];
    pd=positions.start;
    pd_p=positions.start_p;
    during:
    trajectory_update = 0;
  state NO_VALID_BALL_VALUE
    entry:
    state=3;
  CATCH -> INIT [order 1] : [reset_flow_chart]
  (default) -> INIT
  NO_VALID_BALL_VALUE -> INIT [order 1] : [reset_flow_chart]
  INIT_GOTO_START -> INIT [order 1] : [reset_flow_chart]
  GO_TO_START_FROM_NO_CATCH -> INIT [order 1] : [reset_flow_chart]
  READY -> INIT [order 1] : [reset_flow_chart]
  INIT -> INIT_GOTO_START : [init_goto_start && motion_enable]
  INIT_GOTO_START -> READY [order 2] : [after(0.5,sec)]
  READY -> CATCH [order 2] : [isBallValueValid(point_in)]
  GO_TO_START_FROM_NO_CATCH -> READY [order 2] : [after(0.5,sec)]
  CATCH -> NO_VALID_BALL_VALUE [order 2] : [t_in > t_catch_predict(2)]
  NO_VALID_BALL_VALUE -> GO_TO_START_FROM_NO_CATCH [order 2] : [after(1,sec)]
  data: t_in function_input double size=1; t_start function_input double size=1; point_in function_input double size=3; init function_input double size=1; pd function_output size=3; pd_p function_output size=3; use_pred function_output size=1; t_catch_predict function_output size=[1,2]; pred_update function_output; init_number_of_samples function_input double size=1; valid function_output size=1; data_point function_input size=3; state output; t_in input; point_in input; pd output; pd_p output; t_catch_predict output; use_pred output; positions parameter; t_start output; init_goto_start input; reset_flow_chart input; trajectory_update output; init_number_of_samples input; motion_enable input
  function valid  = isBallValueValid(data_point):
    | function valid  = isBallValueValid(data_point)
    | valid = ~(data_point(1) == 0 && data_point(2) == 0 && data_point(3) == 0);

== matlab function controller_ballcatcher_overdo/Robot Pose Logger ==
  data: application_button input; robot_model input
function fcn(application_button,robot_model)
  persistent last_application_button;

  if(isempty(last_application_button))
    last_application_button=application_button;
  end
  
  if(last_application_button~=application_button && application_button)
    fprintf('[%.10f,%.10f,%.10f,%.10f;%.10f,%.10f,%.10f,%.10f;%.10f,%.10f,%.10f,%.10f],...',...
      robot_model.H(1,1),robot_model.H(1,2),robot_model.H(1,3),robot_model.H(1,4),...
      robot_model.H(2,1),robot_model.H(2,2),robot_model.H(2,3),robot_model.H(2,4),...
      robot_model.H(3,1),robot_model.H(3,2),robot_model.H(3,3),robot_model.H(3,4));
  end
  
  last_application_button=application_button;
end

== matlab function controller_ballcatcher_overdo/Sensor Filters/f_tau_slow ==
  data: u input; tau_slow output; param_controller parameter; filter_tau_slow_T_1 parameter
function tau_slow = func(u,param_controller, filter_tau_slow_T_1)
  persistent x;
  
  T_1=filter_tau_slow_T_1;
  alpha=exp(-param_controller.T_a./T_1);
  if(isempty(x))
    x=1./(1-alpha).*u;
    tau_slow=u;
  else
    tau_slow=(1-alpha).*x;
    x=alpha.*x+u;
  end
end

== matlab function controller_ballcatcher_overdo/Rigid Body Controller/Gravitation compensation q-based/Gravitation compensation q-based ==
  data: robot_model input; tau_d output; K_D input; slope_factor input; param_nullspace parameter; barrier output; param_robot parameter
function [tau_d,barrier] = fcn(robot_model, K_D,slope_factor,param_nullspace,param_robot)
  n=param_robot.n;
  %% Barrier or penalty functions for nullspace controller
  %Desired position for nullspace
  p_1=...
    slope_factor*param_nullspace.q_limit_slope(1:n)./...
      (1./(param_nullspace.q_limit_range(1:n).^2)...
      -1./((param_nullspace.q_limit_upper(1:n)-param_nullspace.q_limit_lower(1:n)-param_nullspace.q_limit_range(1:n)).^2));
    
  q=robot_model.q;
  barrier=zeros(size(q));
  valid=q<param_nullspace.q_limit_upper(1:n) & q>param_nullspace.q_limit_lower(1:n);
  inside=q<(param_nullspace.q_limit_upper(1:n)-param_nullspace.q_limit_range(1:n)) & ...
    q>(param_nullspace.q_limit_lower(1:n)+param_nullspace.q_limit_range(1:n));
  barrier(valid)=(1./(q(valid)-param_nullspace.q_limit_upper(valid)).^2 ...
      -1./(param_nullspace.q_limit_lower(valid)-q(valid)).^2).*p_1(valid)...
    -slope_factor*param_nullspace.q_limit_slope(valid).*sign(q(valid));
  barrier(~valid)=NaN;
  barrier(inside)=0;
  
  tau_d=robot_model.g-K_D*robot_model.q_p-barrier;
end

== matlab function controller_ballcatcher_overdo/Sensor Filters/f_theta_p ==
  data: u input; theta_p output; filter_theta_p_T_1 parameter; param_controller parameter
function theta_p = func(u,filter_theta_p_T_1,param_controller)
  persistent x;
  
  T_1=filter_theta_p_T_1;
  V=1/param_controller.T_a*(1-exp(-param_controller.T_a./T_1));
  if(isempty(x))
    x=-V.*u;
    theta_p=zeros(size(u));
  else
    theta_p=x+V.*u;
    x=exp(-param_controller.T_a./T_1).*x+(exp(-param_controller.T_a./T_1)-1).*V.*u;
  end
end

== matlab function controller_ballcatcher_overdo/Rigid Body Controller/Joint-based E//A Linearization/Joint-based E//A Linearization ==
  data: q_d input; robot_model input; motion_enabled input; tau_d output; param_robot parameter; controller input; param_controller parameter; e output; e_p output
function [tau_d,e,e_p] = fcn(q_d,robot_model,motion_enabled, param_robot,controller,param_controller)
  persistent e_I;
  
  if(~motion_enabled || isempty(e_I))
    e_I=zeros(param_robot.n,1);
  end
  
  q_pp_d=q_d(2*param_robot.n+1:3*param_robot.n);
  q_p_d=q_d(param_robot.n+1:2*param_robot.n);
  q_d=q_d(1:param_robot.n);
  
  K_I=controller(1)*ones(param_robot.n,1);
  K_0=controller(2)*ones(param_robot.n,1);
  K_1=controller(3)*ones(param_robot.n,1);
  
  q=robot_model.q;
  q_p=robot_model.q_p;
  
  %Common "Computed Torque" equations
  M=robot_model.M;
  C=robot_model.C;
  g=robot_model.g;
  n=C*q_p+g;

  e=q-q_d;
  e_p=q_p-q_p_d;
  v=q_pp_d-K_1.*e_p-K_0.*e-K_I.*e_I;
  
  tau_d=M*v+n;
  
  e_I=e_I+e*param_controller.T_a;
end

== matlab function controller_ballcatcher_overdo/Robot Model ==
  data: tau input; tau_p input; theta input; robot_model output Bus: robot_model; theta_p input; param_robot parameter; param_controller parameter
function robot_model = fcn(tau,tau_p,theta,theta_p,param_robot,param_controller)
  K=param_robot.K;
  
  robot_model=struct();
  %The calculation of q and q_p has to be performed with consistent cutoff
  %frequencies for the corresponding filters. The filters for q, q_p, tau
  %and tau_p have to have the same cutoff frequency.
  q=theta-diag(K).\tau;
  q_p=theta_p-diag(K).\tau_p;
  robot_model.q=q;
  robot_model.q_p=q_p;
  %Path Following Control with reverse kinematic
  robot_model.H=[iiwa_homogeneous_transformation_endeffector(q,param_robot);[0 0 0 1]];
  robot_model.J=iiwa_jacobian(q,param_robot);
  robot_model.J_p=iiwa_jacobian_p(q,q_p,param_robot);
  %If the singular perturbation controller is selected, the mass matrix has
  %to be modified according to Ott2008, Eq. (5.28).
  robot_model.M=iiwa_reduced_inertia_matrix(q,param_robot);
  %More efficient implementation for M+(I+K_tau)\B with diagonal
  %matrices K_tau and B: Only handle the diagonal elements.
  robot_model.M=robot_model.M+diag((1+param_controller.singular_perturbation.K_tau).\diag(param_robot.B));
  robot_model.C=iiwa_reduced_coriolis_matrix(q,q_p,param_robot);
  robot_model.g=iiwa_gravitational_force(q,param_robot);
end

== matlab function controller_ballcatcher_overdo/Torque Saturation1 ==
  data: tau_in input; tau_out output; param_robot parameter
function tau_out = fcn(tau_in,param_robot)
  
  tau_out = tau_in;

  for i = 1:param_robot.n
     if tau_in(i) > param_robot.tau_saturation_max(i)
        tau_out(i) = param_robot.tau_saturation_max(i);
     elseif tau_in(i) < -param_robot.tau_saturation_max(i)
        tau_out(i) = -param_robot.tau_saturation_max(i);
     end
  end
end
